simulink model "GradientAscent"  (R2020b)
settings: Solver=FixedStepDiscrete  StartTime=0.0  StopTime=150  FixedStep=Ts  RelTol=1e-3
PreLoadFcn:
  | ROSconfig
  | wptsSignalSetup
InitFcn:
  | configParameters
StartFcn:
  | gazeboSetup
StopFcn:
  | gazeboReset
  | goalreset
  | loadResults
model workspace (MAT data in the model file):
  goalpoints = Simulink.Signal
  goalpoints.DataType = 'auto'
  goalpoints.Dimensions = -1
  goalpoints.DimensionsMode = 'auto'
  goalpoints.Complexity = 'auto'
  goalpoints.SampleTime = -1
  goalpoints.SamplingMode = 'auto'
  goals = Simulink.Signal
  goals.DataType = 'auto'
  goals.Dimensions = -1
  goals.DimensionsMode = 'auto'
  goals.Complexity = 'auto'
  goals.SampleTime = -1
  goals.SamplingMode = 'auto'
  idx = 1
  y = Simulink.Parameter
  y.DataType = 'auto'
  y.Dimensions = [0 0]
values from neighbouring files (symbols this model uses):
  distThresh = .875    (= 0.875)    [GradientAscentMetrics.m]
  m = [m; i*(2*pi/M)]    [SensorArrangementPlots.m]    (also in sensorArrayTesting.m = [0;0;1.2566;2.5133;3.7699;5.0265])
  mag = 2    [GradientAscentMetrics.m]
  sensorDist = 1    [GradientAscentMetrics.m]
undefined symbols (not defined in the file or in its folder): angmax, Angular, concDetectionAccuracy, DiscIntNeverNeededParam, distError, get, init, initX, initY, Kd, Ki, Kp, Linear, MaxC, N, n, OffsetY, PlumeD, Res, ResX, ResY, sourceAccuracy, Tmax, vmax, wgain
libraries: simulink x14, dspswit3 x4, robotlib x3, sm_lib x2, dspsnks4 x2, nesl_utility x1, dspindex x1, mobileRoboticsLib x1
PauseFcn:
  | gazeboPause
settings Model: OrderedModelArguments=off  Creator=ty  LastModifiedBy=Tyreeses'
settings SolverCC: AlgebraicLoopSolver=LineSearch
settings DataIOCC: ExternalInput=[r, b]  SaveFormat=Array  SaveState=on  InspectSignalLogs=on  ReturnWorkspaceOutputs=off  StateSaveName=wpts
settings DebuggingCC: ArithmeticOperatorsInVariantConditions=warning
settings SFSimCC: SimUseLocalCustomCode=off  CustomCodeUndefinedFunction=UseInterfaceOnly
settings RTWCC: RTWUseLocalCustomCode=off
settings SimMechanicsCC: VisOnUpdateDiagram=on  VisDuringSimulation=on  DefaultBodyColor=[.877 0 0]
settings ExplorerConfigSet: SimMechanicsOpenEditorOnUpdate=off  InternalSimMechanicsExplorerSettings="<ExplorerConfiguration><canonicalview>default</canonicalview><AnimationSetting><BasePlaybackSpeed>1.0</BasePlaybackSpeed><PlaybackSpeedFactor>4.0</PlaybackSpeedFactor></AnimationSetting><TilePanel><TileInfo><Tiles Columns=\"2\" Count=\"4\" Rows=\"2\"><Column Weight=\"0.5\"/><Column Weight=\"0.5\"/><Row Weight=\"0.5\"/><Row Weight=\"0.5\"/><Tile Height=\"1\" Width=\"1\" X=\"0\" Y=\"0\"/><Tile Height=\"1\" Width=\"1\" X=\"0\" Y=\"1\"/><Tile Height=\"1\" Width=\"1\" X=\"1\" Y=\"0\"/><Tile Height=\"1\" Width=\"1\" X=\"1\" Y=\"1\"/></Tiles></TileInfo><SceneInfo><SceneViewer><BGColor><R>0.60000002384185791</R><G>0.60000002384185791</G><B>0.60000002384185791</B></BGColor><Camera><DoPerspective>off</DoPerspective><Position><X>0.523539858098702515</X><Y>-0.526832295844210763</Y><Z>1.31558763938248235</Z></Position><Center><X>0.523539858098702515</X><Y>-0.526832295844210763</Y><Z>0.315587639382482354</Z></Center><Up><X>0</X><Y>1</Y><Z>-0</Z></Up><ViewLimDist>1</ViewLimDist><YLim>8.09056691591361421</YLim><XLim>11.4549610789668002</XLim></Camera></SceneViewer><SceneViewer><BGColor><R>0.60000002384185791</R><G>0.60000002384185791</G><B>0.60000002384185791</B></BGColor><Camera><DoPerspective>off</DoPerspective><Position><X>-1.00000000034924597</X><Y>-0.123102183445061519</Y><Z>0.275798201199813964</Z></Position><Center><X>-3.49245965480804443e-10</X><Y>-0.123102183445061519</Y><Z>0.275798201199813964</Z></Center><Up><X>0</X><Y>0</Y><Z>1</Z></Up><ViewLimDist>1</ViewLimDist><YLim>3.47753295219900371</YLim><XLim>4.92363576400452985</XLim></Camera></SceneViewer><SceneViewer><BGColor><R>0.60000002384185791</R><G>0.60000002384185791</G><B>0.60000002384185791</B></BGColor><Camera><DoPerspective>off</DoPerspective><Position><X>0.692144908773628886</X><Y>-0.692774488443842151</Y><Z>0.641997243049143074</Z></Position><Center><X>0.114794639584003433</X><Y>-0.115424219254216046</Y><Z>0.0646469738595174259</Z></Center><Up><X>-0.408248290463863073</X><Y>0.408248290463863073</Y><Z>0.816496580927726145</Z></Up><ViewLimDist>1</ViewLimDist><YLim>6.0070720394774666</YLim><XLim>8.50506239252750262</XLim></Camera></SceneViewer><SceneViewer><BGColor><R>0.60000002384185791</R><G>0.60000002384185791</G><B>0.60000002384185791</B></BGColor><Camera><DoPerspective>off</DoPerspective><Position><X>0.0489598554332313918</X><Y>-0.287272213681231237</Y><Z>1.31558770067272501</Z></Position><Center><X>0.0489598554332313918</X><Y>-0.287272213681231237</Y><Z>0.315587700672725013</Z></Center><Up><X>0</X><Y>1</Y><Z>-0</Z></Up><ViewLimDist>1</ViewLimDist><YLim>2.42704539801906094</YLim><XLim>3.4363118011556999</XLim></Camera></SceneViewer></SceneInfo></TilePanel><MechEditorPanel><Cameras><Camera><Id>Camera1</Id><Value><Name>TopCamera1</Name><NativeCamera><PositionKeyframeSet><Keyframe><Time>+0.0000000000000000e+00</Time><Value><X>+2.1442706964244174e-01</X><Y>+2.3082412087368320e-01</Y><Z>+8.5801428178680403e+00</Z></Value></Keyframe></PositionKeyframeSet><CenterKeyframeSet><Keyframe><Time>+0.0000000000000000e+00</Time><Value><X>+1.7666087274208450e-01</X><Y>+1.6219238056249624e-01</Y><Z>+3.9566976367888529e-01</Z></Value></Keyframe></CenterKeyframeSet><UpVectorKeyframeSet><Keyframe><Time>+0.0000000000000000e+00</Time><Value><X>-1.4536948631457236e-02</X><Y>+9.9985973958876295e-01</Y><Z>-8.3173477730344968e-03</Z></Value></Keyframe></UpVectorKeyframeSet></NativeCamera></Value></Camera></Cameras><GfxPanelCameraMap/><VideoCreator><PlaybackSpeedRatio>1.0</PlaybackSpeedRatio><FrameRate>30</FrameRate><VideoFormat>Motion JPEG AVI</VideoFormat><FrameSize>auto</FrameSize></VideoCreator></MechEditorPanel></ExplorerConfiguration>"

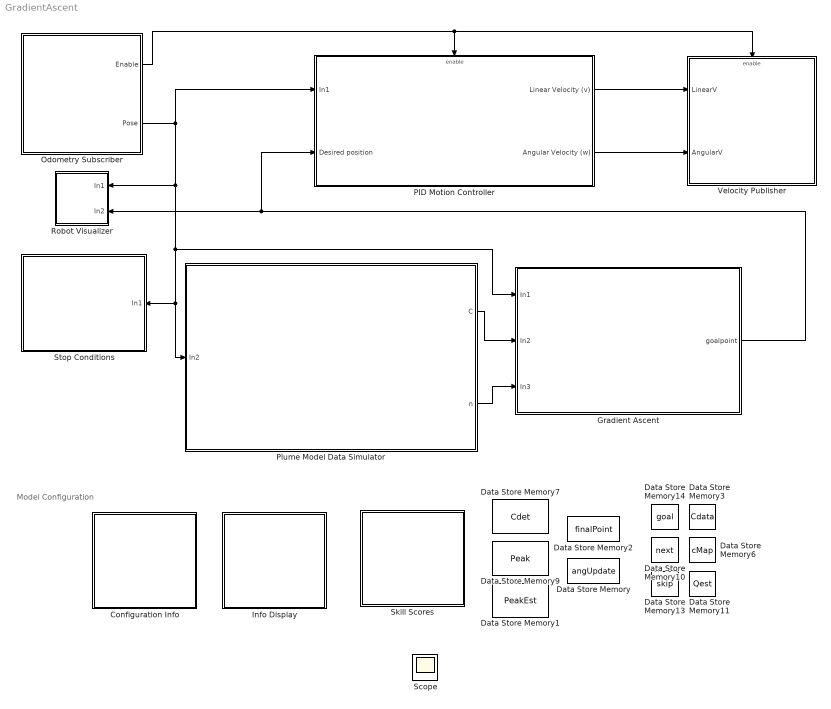
== system GradientAscent ==
  note: Model Configuration
  Configuration Info : Subsystem
  Data Store Memory : DataStoreMemory  DataStoreName=angUpdate  ReadBeforeWriteMsg=warning  WriteAfterWriteMsg=warning  WriteAfterReadMsg=warning  ShowAdditionalParam=off
  Data Store Memory1 : DataStoreMemory  DataStoreName=PeakEst  ReadBeforeWriteMsg=warning  WriteAfterWriteMsg=warning  WriteAfterReadMsg=warning  InitialValue=[(initX) (initY)]  VectorParams1D=off  ShowAdditionalParam=off
  Data Store Memory10 : DataStoreMemory  DataStoreName=next  ReadBeforeWriteMsg=warning  WriteAfterWriteMsg=warning  WriteAfterReadMsg=warning  ShowAdditionalParam=off
  Data Store Memory11 : DataStoreMemory  DataStoreName=Qest  ReadBeforeWriteMsg=warning  WriteAfterWriteMsg=warning  WriteAfterReadMsg=warning  ShowAdditionalParam=off
  Data Store Memory13 : DataStoreMemory  DataStoreName=skip  ReadBeforeWriteMsg=warning  WriteAfterWriteMsg=warning  WriteAfterReadMsg=warning  ShowAdditionalParam=off
  Data Store Memory14 : DataStoreMemory  DataStoreName=goal  ReadBeforeWriteMsg=warning  WriteAfterWriteMsg=warning  WriteAfterReadMsg=warning  VectorParams1D=off  ShowAdditionalParam=off
  Data Store Memory2 : DataStoreMemory  DataStoreName=finalPoint  ReadBeforeWriteMsg=warning  WriteAfterWriteMsg=warning  WriteAfterReadMsg=warning  ShowAdditionalParam=off
  Data Store Memory3 : DataStoreMemory  DataStoreName=Cdata  ReadBeforeWriteMsg=warning  WriteAfterWriteMsg=warning  WriteAfterReadMsg=warning  InitialValue=ones(N+1,1)  ShowAdditionalParam=off  OutDataTypeStr=double
  Data Store Memory6 : DataStoreMemory  DataStoreName=cMap  ReadBeforeWriteMsg=warning  WriteAfterWriteMsg=warning  WriteAfterReadMsg=warning  InitialValue=zeros(50,500)  VectorParams1D=off  ShowAdditionalParam=off
  Data Store Memory7 : DataStoreMemory  DataStoreName=Cdet  ReadBeforeWriteMsg=warning  WriteAfterWriteMsg=warning  WriteAfterReadMsg=warning  ShowAdditionalParam=off
  Data Store Memory9 : DataStoreMemory  DataStoreName=Peak  ReadBeforeWriteMsg=warning  WriteAfterWriteMsg=warning  WriteAfterReadMsg=warning  InitialValue=[0 0]  ShowAdditionalParam=off
  Gradient Ascent : Subsystem
  Info Display : Subsystem
  Odometry Subscriber : Subsystem
  PID Motion Controller : Subsystem
  Plume Model Data Simulator : Subsystem
  Robot Visualizer : Subsystem
  Skill Scores : Subsystem
  Stop Conditions : Subsystem
  Velocity Publisher : Subsystem
  Scope : Scope
  wires:
  Odometry Subscriber/1(Enable) -> Velocity Publisher/Enable, PID Motion Controller/Enable
  PID Motion Controller/1(Linear Velocity (v)) -> Velocity Publisher/1(LinearV)
  PID Motion Controller/2(Angular Velocity (w)) -> Velocity Publisher/2(AngularV)
  Gradient Ascent/1(goalpoint) -> PID Motion Controller/2(Desired position), Robot Visualizer/2(In2)
  Plume Model Data Simulator/1(C) -> Gradient Ascent/2(In2)
  Plume Model Data Simulator/2(n) -> Gradient Ascent/3(In3)
  Odometry Subscriber/2(Pose) -> Plume Model Data Simulator/1(In2), Stop Conditions/1(In1), Gradient Ascent/1(In1), Robot Visualizer/1(In1), PID Motion Controller/1(In1)

== system GradientAscent/Configuration Info ==
  note: Nodes :
      | Publishers:
      | /sim_p3at/cmd_vel
      | /toggle_led
      | Subscribers:
      | /sim_p3at/odom
      | Messages:
      | geometry_msgs/Twist
      | std_msgs/Empty
  note: Startup Programs :
      | roscore
      | roslaunch nre_p3at p3at.gazebo.launch (starts Gazebo and /sim_p3at Nodes)
      | Arduino: ledtest3.ino
      | rosrun rosserial_python serial_node.py /dev/ttyACM0
      | MATLAB: (Simulink project)
  note: SS Parameters :
      | Expansion Constant: 2
  note: Plume Parameters :
      |
      | Diffusion constant (m2/s): c_diff = .8
      |
      | Advection velocity values (m/s): ux = 0 uy = 0 uz = 0.2
      |
      | Simulation Time (seconds): T = 10
      |
      | Domain dimensions (meters): L = 50 B = 50 H = 5
  "Counter " : Subsystem  Commented=on
  Floating Scope : Scope  Commented=on
      settings: Floating=on
  MechanismConfiguration : sm_lib/Utilities/Mechanism Configuration  UniformGravity=Constant  GravityVector=[0 0 -9.80665]  GravityUnits=m/s^2  LinearizationDelta=0.01
  Solver Configuration : nesl_utility/Solver Configuration  PhysicalDomain=network_engine_domain  SubClassName=solver  LeftPortType=input  RightPortType=generic  Accelerate=off  Tones=[]  Harmonics=[]  SimulateNoise=off  Profile=off  UseLocalSampling=off  EnableSwitchedLinearOptims=on  FrequencyDomain=off  UseCCode=off  RelTol=0.001  AbsTol=1e-06  MinStep=1e-09  ToWorkspace=off  RevertToSquareIcSolve=off  NumHomotopyIterations=100  PhasorMode=off  PhasorModeNumHarmonics=1  DoDC=on  ResidualTolerance=1e-09  UseLocalSolver=on  LocalSolverChoice=NE_BACKWARD_EULER_ADVANCER  LocalSolverSampleTime=Ts  DoFixedCost=on  MaxNonlinIter=3  MaxModeIter=2  LinearAlgebra=Sparse  DelaysMemoryBudget=1024  AutomaticFiltering=on  FilteringTimeConstant=0.01
  World : sm_lib/Frames and Transforms/World Frame
  connections:
  MechanismConfiguration/RConn1 -- World/RConn1 -- Solver Configuration/RConn1

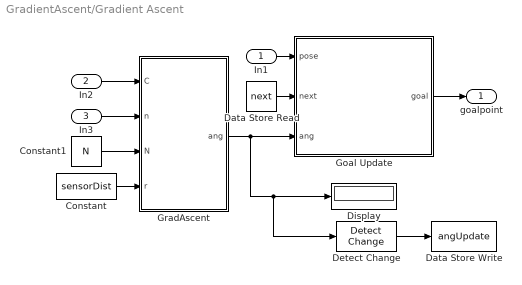
== system GradientAscent/Gradient Ascent ==
  In1 : Inport
  In2 : Inport  Port=2
  In3 : Inport  Port=3
  Constant : Constant  Value=sensorDist
  Constant1 : Constant  Value=N
  Data Store Read : DataStoreRead  DataStoreName=next
  Data Store Write : DataStoreWrite  DataStoreName=angUpdate
  Detect Change : simulink/Logic and Bit Operations/Detect Change  vinit=1.514  OutDataTypeStr=boolean
  Display : Display
  Goal Update : Subsystem
  GradAscent : MATLAB Function  TreatAsAtomicUnit=on
  goalpoint : Outport  VectorParamsAs1DForOutWhenUnconnected=off
  wires:
  In1/1 -> Goal Update/1(pose)
  In3/1 -> GradAscent/2(n)
  GradAscent/1(ang) -> Detect Change/1, Display/1, Goal Update/3(ang)
  Goal Update/1(goal) -> goalpoint/1
  Data Store Read/1 -> Goal Update/2(next)
  Constant/1 -> GradAscent/4(r)
  Constant1/1 -> GradAscent/3(N)
  Detect Change/1 -> Data Store Write/1
  In2/1 -> GradAscent/1(C)

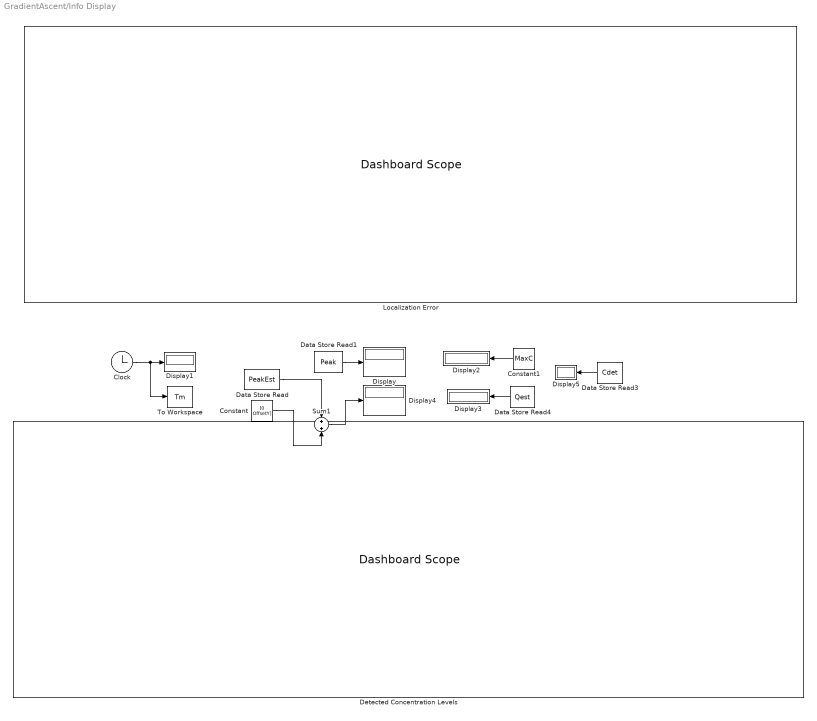
== system GradientAscent/Info Display ==
  Clock : Clock
      settings: Decimation=2
  Constant : Constant  Value=[0 OffsetY]
  Constant1 : Constant  Value=MaxC
  Data Store Read : DataStoreRead  DataStoreName=PeakEst
  Data Store Read1 : DataStoreRead  DataStoreName=Peak
  Data Store Read3 : DataStoreRead  DataStoreName=Cdet
  Data Store Read4 : DataStoreRead  DataStoreName=Qest
  Detected Concentration Levels : DashboardScope  ShowInitialText=off  Ymin=0  Ymax=1000
  Display{,1..5} (6 alike) : Display
  Localization Error : DashboardScope  Ymin=0  Ymax=1.25  LegendPosition=Hide
  Sum1 : Sum
  To Workspace : ToWorkspace  VariableName=Tm  SampleTime=-1
  wires:
  Data Store Read1/1 -> Display/1
  Data Store Read/1 -> Sum1/1
  Data Store Read4/1 -> Display3/1
  Constant1/1 -> Display2/1
  Clock/1 -> To Workspace/1, Display1/1
  Data Store Read3/1 -> Display5/1
  Constant/1 -> Sum1/2
  Sum1/1 -> Display4/1

== system GradientAscent/Odometry Subscriber ==
  Odom Conversion : Subsystem
  Subscribe1 : robotlib/Subscribe  topicSource=Select from ROS network  topic=/sim_p3at/odom  messageType=nav_msgs/Odometry  SampleTime=-1  legacyBusStruct=off  messageQueueLength=51
  Enable : Outport  VectorParamsAs1DForOutWhenUnconnected=off
  Pose : Outport  Port=2  VectorParamsAs1DForOutWhenUnconnected=off
  wires:
  Subscribe1/1 -> Enable/1
  Subscribe1/2 -> Odom Conversion/1(In1)
  Odom Conversion/1(pose) -> Pose/1

== system GradientAscent/PID Motion Controller ==
  In1 : Inport
  Desired position : Inport  Port=2
  Enable : EnablePort
  Constant3 : Constant  Value=0
  Demux : Demux  Outputs=3
  PID Calculations : Subsystem
  Switch1 : Switch  Criteria=u2 ~= 0
  Linear Velocity (v) : Outport  VectorParamsAs1DForOutWhenUnconnected=off
  Angular Velocity (w) : Outport  Port=2  VectorParamsAs1DForOutWhenUnconnected=off
  wires:
  Switch1/1 -> Angular Velocity (w)/1
  Constant3/1 -> Switch1/1
  Demux/1 -> PID Calculations/3(x)
  Demux/2 -> PID Calculations/2(y)
  Demux/3 -> PID Calculations/4(theta)
  PID Calculations/3(w) -> Switch1/3
  In1/1 -> Demux/1
  PID Calculations/2(next) -> Switch1/2
  Desired position/1 -> PID Calculations/1(SP)  "SP"
  PID Calculations/1(v) -> Linear Velocity (v)/1

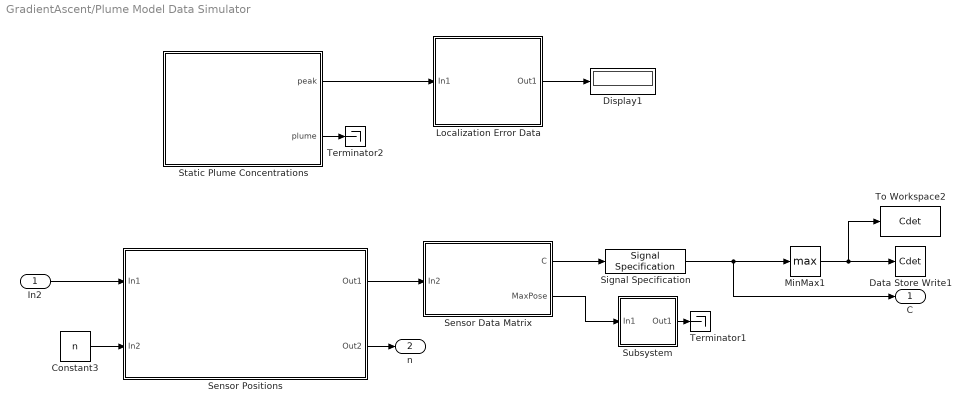
== system GradientAscent/Plume Model Data Simulator ==
  In2 : Inport
  Constant3 : Constant  Value=n
  Data Store Write1 : DataStoreWrite  DataStoreName=Cdet
  Display1 : Display
  Localization Error Data : Subsystem
  MinMax1 : MinMax  Function=max
  Sensor Data Matrix : Subsystem
  Sensor Positions : Subsystem
  Signal Specification : SignalSpecification  OutDataTypeStr=double  SampleTime=.01
  Static Plume Concentrations : Subsystem
  Subsystem : Subsystem
  Terminator1 : Terminator
  Terminator2 : Terminator
  To Workspace2 : ToWorkspace  VariableName=Cdet  SaveFormat=Timeseries  SampleTime=-1
  C : Outport  VectorParamsAs1DForOutWhenUnconnected=off
  n : Outport  Port=2  VectorParamsAs1DForOutWhenUnconnected=off
  wires:
  Sensor Positions/1(Out1) -> Sensor Data Matrix/1(In2)
  MinMax1/1 -> To Workspace2/1, Data Store Write1/1
  Sensor Data Matrix/1(C) -> Signal Specification/1
  Signal Specification/1 -> C/1, MinMax1/1
  In2/1 -> Sensor Positions/1(In1)
  Constant3/1 -> Sensor Positions/2(In2)
  Static Plume Concentrations/1(peak) -> Localization Error Data/1(In1)
  Static Plume Concentrations/2(plume) -> Terminator2/1
  Localization Error Data/1(Out1) -> Display1/1
  Sensor Data Matrix/2(MaxPose) -> Subsystem/1(In1)
  Subsystem/1(Out1) -> Terminator1/1
  Sensor Positions/2(Out2) -> n/1

== system GradientAscent/Robot Visualizer ==
  In1 : Inport
  In2 : Inport  Port=2
  Constant1 : Constant
  Current Origin : dspindex/Variable Selector  NumInputs=1  rowsOrCols=Rows  IdxMode=Variable  Elements=[1 3]  ZerOneIdxMode=One-based  errmode=Clip Index  FillMode=off  FillValues=0
  Data Store Read : DataStoreRead  DataStoreName=next
  Data Store Write : DataStoreWrite  DataStoreName=PeakEst
  Robot Visualizer : mobileRoboticsLib/Environments/Robot Visualizer  Priority=99  robotRadius=.34  mapName=gasMap  showTrajectory=on  hasWaypoints=on  hasLidar=off  sensorOffset=[ 0 0 ]  scanAngles=0  hasObjDetector=off  objDetectorOffset=[ 0,0 ]  objDetectorAngle=0  objDetectorFOV=0  objDetectorMaxRange=0  objectColors=[1,0,0;0,1,0;0,0,1]  objectMarkers='s'
  To Workspace : ToWorkspace  VariableName=goalpoints  SampleTime=-1
      settings: Save2DSignal=2-D array (concatenate along first dimension)
  Triggered To Workspace : dspsnks4/Triggered To Workspace  TriggerType=Rising edge  VariableName=pathUpdates  Buffer=1000  Save2DMode=3-D array (concatenate along third dimension)
      settings: SourceProductBaseCode=DS  FixptAsFi=off
  wires:
  In1/1 -> Robot Visualizer/1
  In2/1 -> To Workspace/1, Current Origin/1, Data Store Write/1, Robot Visualizer/2
  Data Store Read/1 -> Triggered To Workspace/Trigger
  Constant1/1 -> Current Origin/2
  Current Origin/1 -> Triggered To Workspace/1

== system GradientAscent/Skill Scores ==
  Location Estimate (SL) : Subsystem
  Source Estimate (SQ) : Subsystem

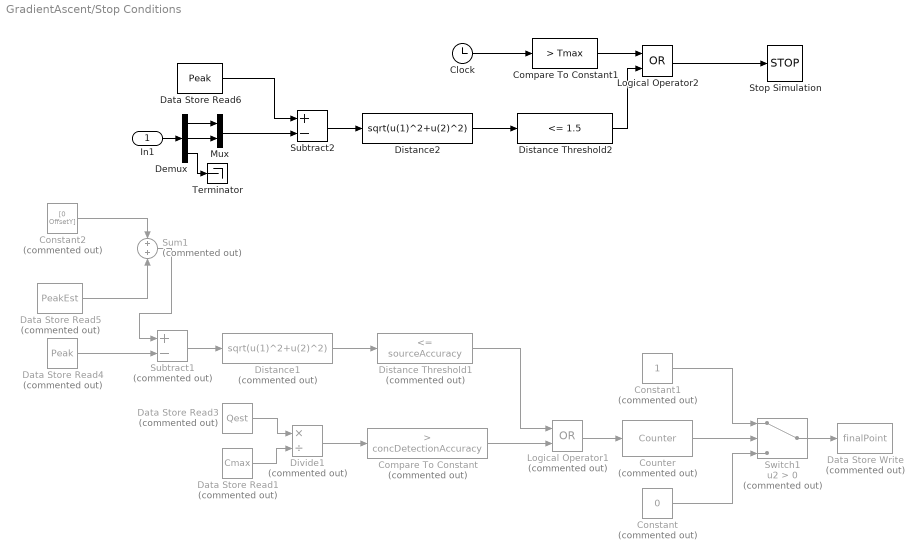
== system GradientAscent/Stop Conditions ==
  In1 : Inport
  Clock : Clock
  Compare To Constant : simulink/Logic and Bit Operations/Compare To Constant  Commented=on  relop=>  const=concDetectionAccuracy  OutDataTypeStr=boolean
  Compare To Constant1 : simulink/Logic and Bit Operations/Compare To Constant  relop=>  const=Tmax  OutDataTypeStr=boolean
  Constant : Constant  Commented=on  Value=0
  Constant1 : Constant  Commented=on
  Constant2 : Constant  Commented=on  Value=[0 OffsetY]
  Counter : dspswit3/Counter  Commented=on  Direction=Up  CountEvent=Rising edge  CounterSize=User defined  MaxCount=255  InitialCount=0  Output=Count  HitValue=32  ResetInput=off  SamplesPerFrame=1  Ts=1  CntDtype=double  HitDtype=Logical
  Data Store Read1 : DataStoreRead  Commented=on  DataStoreName=Cmax
  Data Store Read3 : DataStoreRead  Commented=on  DataStoreName=Qest
  Data Store Read4 : DataStoreRead  Commented=on  DataStoreName=Peak
  Data Store Read5 : DataStoreRead  Commented=on  DataStoreName=PeakEst
  Data Store Read6 : DataStoreRead  DataStoreName=Peak
  Data Store Write : DataStoreWrite  Commented=on  DataStoreName=finalPoint
  Demux : Demux  Outputs=3
  Distance Threshold1 : simulink/Logic and Bit Operations/Compare To Constant  Commented=on  relop=<=  const=sourceAccuracy  OutDataTypeStr=boolean
  Distance Threshold2 : simulink/Logic and Bit Operations/Compare To Constant  relop=<=  const=1.5  OutDataTypeStr=boolean
  Distance1 : Fcn  Commented=on  Expr=sqrt(u(1)^2+u(2)^2)
  Distance2 : Fcn  Expr=sqrt(u(1)^2+u(2)^2)
  Divide1 : Product  Commented=on  Inputs=*/
  Logical Operator1 : Logic  Commented=on  Operator=OR  AllPortsSameDT=off  OutDataTypeStr=boolean
  Logical Operator2 : Logic  Operator=OR  AllPortsSameDT=off  OutDataTypeStr=boolean
  Mux : Mux  Inputs=2
  Stop Simulation : Stop
  Subtract1 : Sum  Commented=on  Inputs=+-
  Subtract2 : Sum  Inputs=+-
  Sum1 : Sum  Commented=on
  Switch1 : Switch  Commented=on  Criteria=u2 > Threshold
  Terminator : Terminator
  wires:
  Logical Operator1/1 -> Counter/1
  Compare To Constant/1 -> Logical Operator1/2
  Data Store Read3/1 -> Divide1/1
  Data Store Read5/1 -> Sum1/2
  Subtract1/1 -> Distance1/1
  Distance Threshold1/1 -> Logical Operator1/1
  Data Store Read4/1 -> Subtract1/2
  Data Store Read1/1 -> Divide1/2
  Distance1/1 -> Distance Threshold1/1
  Divide1/1 -> Compare To Constant/1
  Data Store Read6/1 -> Subtract2/1
  Subtract2/1 -> Distance2/1
  Distance2/1 -> Distance Threshold2/1
  Distance Threshold2/1 -> Logical Operator2/2
  Constant1/1 -> Switch1/1
  Constant/1 -> Switch1/3
  Counter/1 -> Switch1/2
  Switch1/1 -> Data Store Write/1
  In1/1 -> Demux/1
  Demux/1 -> Mux/1
  Demux/2 -> Mux/2
  Mux/1 -> Subtract2/2
  Demux/3 -> Terminator/1
  Constant2/1 -> Sum1/1
  Sum1/1 -> Subtract1/1
  Compare To Constant1/1 -> Logical Operator2/1
  Clock/1 -> Compare To Constant1/1
  Logical Operator2/1 -> Stop Simulation/1

== system GradientAscent/Velocity Publisher ==
  LinearV : Inport
  AngularV : Inport  Port=2
  Enable : EnablePort
  Blank Message : robotlib/Blank Message  SourceLibraryInfo=This block requires Robotics System Toolbox  messageType=geometry_msgs/Twist  SampleTime=-1
  Bus Assignment : BusAssignment  DialogController=Simulink.DDGSource_BusAssignment  AssignedSignals=Linear.X,Angular.Z
  Publish1 : robotlib/Publish  SourceLibraryInfo=This block requires Robotics System Toolbox  topicSource=Select from ROS network  topic=/sim_p3at/cmd_vel  messageType=geometry_msgs/Twist  messageQueueLength=105
  wires:
  AngularV/1 -> Bus Assignment/3
  Bus Assignment/1 -> Publish1/1
  LinearV/1 -> Bus Assignment/2
  Blank Message/1 -> Bus Assignment/1

== system GradientAscent/Configuration Info/Counter  ==
  In1 : Inport
  Counter : dspswit3/Counter  Direction=Up  CountEvent=Non-zero sample  CounterSize=User defined  MaxCount=255  InitialCount=0  Output=Count  HitValue=32  ResetInput=off  SamplesPerFrame=1  Ts=1  CntDtype=single  HitDtype=Logical
  Counter1 : dspswit3/Counter  Direction=Up  CountEvent=Rising edge  CounterSize=User defined  MaxCount=255  InitialCount=0  Output=Count  HitValue=32  ResetInput=off  SamplesPerFrame=1  Ts=1  CntDtype=double  HitDtype=Logical
  Detect Increase : simulink/Logic and Bit Operations/Detect Increase  vinit=0.0  OutDataTypeStr=boolean
  Out1 : Outport  VectorParamsAs1DForOutWhenUnconnected=off
  wires:
  In1/1 -> Counter/1
  Counter/1 -> Detect Increase/1
  Detect Increase/1 -> Counter1/1
  Counter1/1 -> Out1/1

== system GradientAscent/Gradient Ascent/Goal Update ==
  pose : Inport
  next : Inport  Port=2
  ang : Inport  Port=3
  Goal Update : Subsystem
  Goal Update Conditions : Subsystem
  Initialize Goal : Subsystem
  Skip Conditions : Subsystem
  goal : Outport  VectorParamsAs1DForOutWhenUnconnected=off
  wires:
  pose/1 -> Goal Update/1(In2)
  ang/1 -> Goal Update/2(In3)
  Goal Update Conditions/1(Out1) -> Goal Update/Enable
  next/1 -> Skip Conditions/1(In1)
  Initialize Goal/1(goal) -> Goal Update Conditions/1(In1), goal/1
  Goal Update/1(Out2) -> Initialize Goal/1(In1)

== system GradientAscent/Odometry Subscriber/Odom Conversion ==
  In1 : Inport
  Bus Selector3 : BusSelector  OutputSignals=Pose.Pose.Position.X,Pose.Pose.Position.Y,Pose.Pose.Orientation.X,Pose.Pose.Orientation.Y,Pose.Pose.Orientation.Z,Pose.Pose.Orientation.W
  Conversion : MATLAB Function  TreatAsAtomicUnit=on
  Mux : Mux  Inputs=3
  pose : Outport  VectorParamsAs1DForOutWhenUnconnected=off
  wires:
  In1/1 -> Bus Selector3/1
  Bus Selector3/3 -> Conversion/1(x)  "<X>"
  Bus Selector3/4 -> Conversion/2(y)  "<Y>"
  Bus Selector3/5 -> Conversion/3(z)  "<Z>"
  Bus Selector3/6 -> Conversion/4(w)  "<W>"
  Bus Selector3/2 -> Mux/2  "<Y>"
  Bus Selector3/1 -> Mux/1  "<X>"
  Mux/1 -> pose/1  "pose"
  Conversion/1(yaw) -> Mux/3

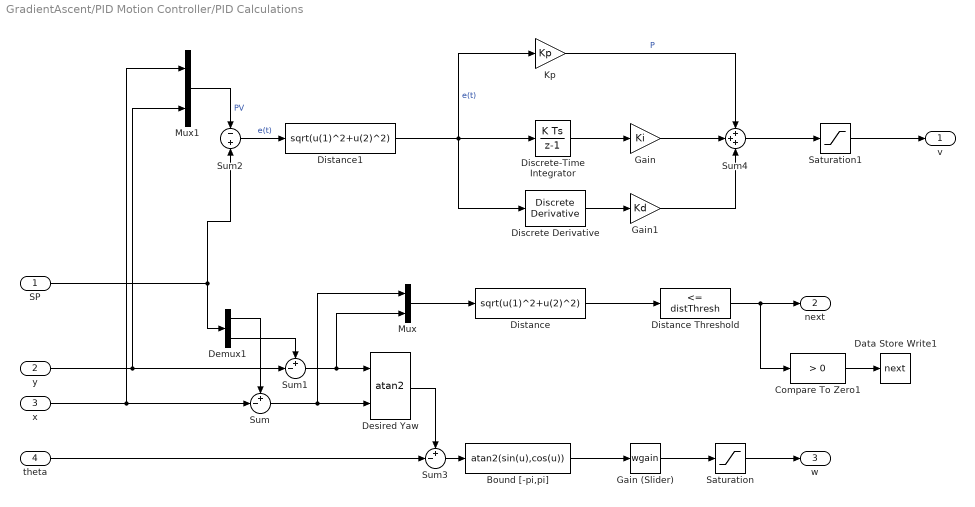
== system GradientAscent/PID Motion Controller/PID Calculations ==
  SP : Inport
  y : Inport  Port=2
  x : Inport  Port=3
  theta : Inport  Port=4
  Bound [-pi,pi] : Fcn  Expr=atan2(sin(u),cos(u))
  Compare To Zero1 : simulink/Logic and Bit Operations/Compare To Zero  relop=>  OutDataTypeStr=boolean
  Data Store Write1 : DataStoreWrite  DataStoreName=next
  Demux1 : Demux  Outputs=2
  Desired Yaw : Trigonometry  Operator=atan2
  Discrete Derivative : simulink/Discrete/Discrete Derivative  gainval=1  ICPrevScaledInput=0.0  OutMin=[]  OutMax=[]  OutDataType=fixdt(1, 16)  OutScaling=2^-10  DoSatur=off
  Discrete-Time Integrator : DiscreteIntegrator  gainval=1  SampleTime=-1  ICPrevOutput=DiscIntNeverNeededParam  ICPrevScaledInput=DiscIntNeverNeededParam
  Distance : Fcn  Expr=sqrt(u(1)^2+u(2)^2)
  Distance Threshold : simulink/Logic and Bit Operations/Compare To Constant  relop=<=  const=distThresh  OutDataTypeStr=boolean
  Distance1 : Fcn  Expr=sqrt(u(1)^2+u(2)^2)
  Gain : Gain  Gain=Ki
  Gain (Slider) : simulink/Math Operations/Slider Gain  gain=wgain  low=1  high=10
  Gain1 : Gain  Gain=Kd
  Kp : Gain  Gain=Kp
  Mux : Mux  Inputs=2
  Mux1 : Mux  Inputs=2
  Saturation : Saturate  UpperLimit=angmax  LowerLimit=-angmax
  Saturation1 : Saturate  UpperLimit=vmax  LowerLimit=-.5
  Sum : Sum  Inputs=+-|
  Sum1 : Sum  Inputs=+-|
  Sum2 : Sum  Inputs=-+
  Sum3 : Sum  Inputs=+-|
  Sum4 : Sum  Inputs=+++
  v : Outport  VectorParamsAs1DForOutWhenUnconnected=off
  next : Outport  Port=2  VectorParamsAs1DForOutWhenUnconnected=off
  w : Outport  Port=3  VectorParamsAs1DForOutWhenUnconnected=off
  wires:
  theta/1 -> Sum3/2
  Desired Yaw/1 -> Sum3/1
  Sum/1 -> Desired Yaw/2, Mux/1
  Gain (Slider)/1 -> Saturation/1
  Saturation/1 -> w/1
  Sum3/1 -> Bound [-pi,pi]/1
  Mux1/1 -> Sum2/1  "PV"
  Kp/1 -> Sum4/1  "P"
  Distance1/1 -> Kp/1, Discrete-Time Integrator/1, Discrete Derivative/1  "e(t)"
  Discrete-Time Integrator/1 -> Gain/1
  Demux1/1 -> Sum/1
  Demux1/2 -> Sum1/1
  Sum1/1 -> Desired Yaw/1, Mux/2
  SP/1 -> Demux1/1, Sum2/2
  y/1 -> Mux1/2, Sum1/2
  x/1 -> Mux1/1, Sum/2
  Distance/1 -> Distance Threshold/1
  Mux/1 -> Distance/1
  Bound [-pi,pi]/1 -> Gain (Slider)/1
  Sum2/1 -> Distance1/1  "e(t)"
  Gain/1 -> Sum4/2
  Sum4/1 -> Saturation1/1
  Discrete Derivative/1 -> Gain1/1
  Gain1/1 -> Sum4/3
  Saturation1/1 -> v/1
  Distance Threshold/1 -> Compare To Zero1/1, next/1
  Compare To Zero1/1 -> Data Store Write1/1

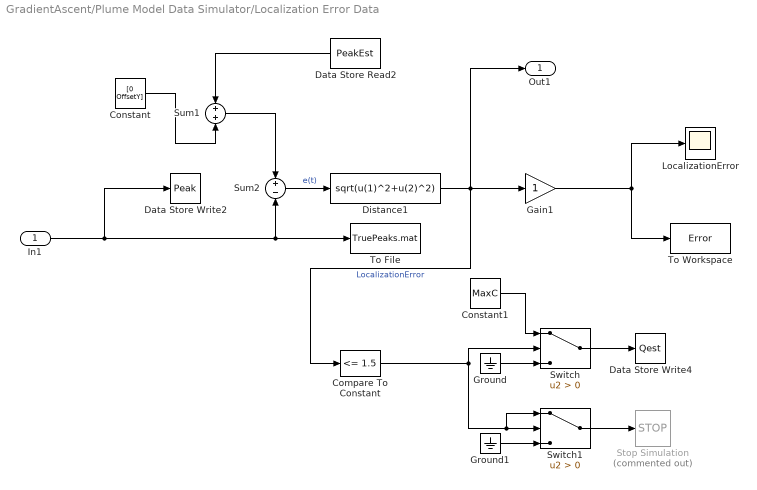
== system GradientAscent/Plume Model Data Simulator/Localization Error Data ==
  In1 : Inport
  Compare To Constant : simulink/Logic and Bit Operations/Compare To Constant  relop=<=  const=1.5  OutDataTypeStr=boolean
  Constant : Constant  Value=[0 OffsetY]
  Constant1 : Constant  Value=MaxC
  Data Store Read2 : DataStoreRead  DataStoreName=PeakEst
  Data Store Write2 : DataStoreWrite  DataStoreName=Peak
  Data Store Write4 : DataStoreWrite  DataStoreName=Qest
  Distance1 : Fcn  Expr=sqrt(u(1)^2+u(2)^2)
  Gain1 : Gain
  Ground : Ground
  Ground1 : Ground
  LocalizationError : Scope
  Stop Simulation : Stop  Commented=on
  Sum1 : Sum
  Sum2 : Sum  Inputs=+-
  Switch : Switch  Criteria=u2 > Threshold
  Switch1 : Switch  Criteria=u2 > Threshold
  To File : ToFile  Filename=TruePeaks.mat  MatrixName=ActualPeaks
      settings: Decimation=2
  To Workspace : ToWorkspace  VariableName=Error  SaveFormat=Timeseries  SampleTime=-1
  Out1 : Outport  VectorParamsAs1DForOutWhenUnconnected=off
  wires:
  Sum2/1 -> Distance1/1  "e(t)"
  Data Store Read2/1 -> Sum1/1
  Distance1/1 -> Out1/1, Compare To Constant/1, Gain1/1  "LocalizationError"
  In1/1 -> Data Store Write2/1, To File/1, Sum2/2
  Constant/1 -> Sum1/2
  Sum1/1 -> Sum2/1
  Gain1/1 -> To Workspace/1, LocalizationError/1
  Compare To Constant/1 -> Switch1/1, Switch1/2, Switch/2
  Ground/1 -> Switch/3
  Constant1/1 -> Switch/1
  Ground1/1 -> Switch1/3
  Switch1/1 -> Stop Simulation/1
  Switch/1 -> Data Store Write4/1

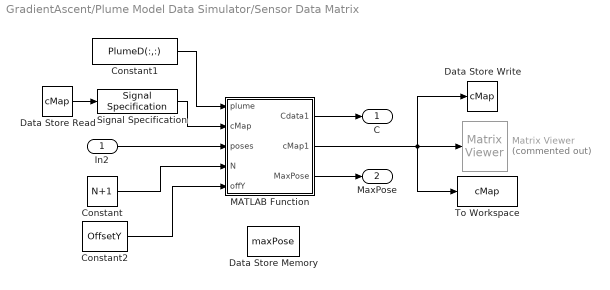
== system GradientAscent/Plume Model Data Simulator/Sensor Data Matrix ==
  In2 : Inport
  Constant : Constant  Value=N+1
  Constant1 : Constant  Value=PlumeD(:,:)
  Constant2 : Constant  Value=OffsetY
  Data Store Memory : DataStoreMemory  DataStoreName=maxPose  ReadBeforeWriteMsg=warning  WriteAfterWriteMsg=warning  WriteAfterReadMsg=warning  InitialValue=init  VectorParams1D=off  ShowAdditionalParam=off  OutDataTypeStr=double
  Data Store Read : DataStoreRead  DataStoreName=cMap
  Data Store Write : DataStoreWrite  DataStoreName=cMap
  MATLAB Function : MATLAB Function  TreatAsAtomicUnit=on
  Matrix Viewer : dspsnks4/Matrix Viewer  Commented=on  ImageParams=off  CMapStr=jet  AxisColorbar=on  AxisParams=off  AxisOrigin=Lower left corner  AxisTickMode=Auto  XTickRange=[0 150]  YTickRange=[0 50]  XLabel=X-axis  YLabel=Y-axis  ZLabel=Concentration  FigPos=get(0,'defaultfigureposition')  AxisZoom=off
      settings: SourceProductBaseCode=DS  YMin=0  YMax=MaxC
  Signal Specification : SignalSpecification  OutDataTypeStr=double  SampleTime=.01
  To Workspace : ToWorkspace  VariableName=cMap  SampleTime=-1
      settings: MaxDataPoints=100
  C : Outport  VectorParamsAs1DForOutWhenUnconnected=off
  MaxPose : Outport  Port=2  VectorParamsAs1DForOutWhenUnconnected=off
  wires:
  Constant/1 -> MATLAB Function/4(N)
  In2/1 -> MATLAB Function/3(poses)
  MATLAB Function/1(Cdata1) -> C/1
  Constant1/1 -> MATLAB Function/1(plume)
  Constant2/1 -> MATLAB Function/5(offY)
  Data Store Read/1 -> Signal Specification/1
  MATLAB Function/2(cMap1) -> To Workspace/1, Data Store Write/1, Matrix Viewer/1
  Signal Specification/1 -> MATLAB Function/2(cMap)
  MATLAB Function/3(MaxPose) -> MaxPose/1

== system GradientAscent/Plume Model Data Simulator/Sensor Positions ==
  In1 : Inport
  In2 : Inport  Port=2
  Radial Sensors : Subsystem
  Sensor Array : Subsystem
  Sensor Center : Subsystem
  Out1 : Outport  VectorParamsAs1DForOutWhenUnconnected=off
  Out2 : Outport  Port=2  VectorParamsAs1DForOutWhenUnconnected=off
  wires:
  In1/1 -> Radial Sensors/1(In1), Sensor Center/1(In2)
  In2/1 -> Radial Sensors/2(In2)
  Sensor Center/1(n) -> Sensor Array/1(In1)
  Sensor Center/2(Out1) -> Sensor Array/2(In2)
  Radial Sensors/1(Out1) -> Sensor Array/3(In3)
  Radial Sensors/2(Out2) -> Sensor Array/4(In4)
  Sensor Array/1(Out2) -> Out1/1
  Sensor Array/2(Out3) -> Out2/1

== system GradientAscent/Plume Model Data Simulator/Static Plume Concentrations ==
  Constant : Constant  Value=OffsetY
  Dynamic Plume Concentration Data : Constant  Value=PlumeD  VectorParams1D=off  OutDataTypeStr=double  LockScale=on
  MATLAB Function : MATLAB Function  TreatAsAtomicUnit=on
  Permute Dimensions1 : PermuteDimensions
  peak : Outport  VectorParamsAs1DForOutWhenUnconnected=off
  plume : Outport  Port=2  VectorParamsAs1DForOutWhenUnconnected=off
  wires:
  Dynamic Plume Concentration Data/1 -> MATLAB Function/1(PlumeD)
  MATLAB Function/1(Plume) -> Permute Dimensions1/1
  Permute Dimensions1/1 -> plume/1
  MATLAB Function/2(Peak) -> peak/1
  Constant/1 -> MATLAB Function/2(OffsetY)

== system GradientAscent/Plume Model Data Simulator/Subsystem ==
  In1 : Inport
  Constant : Constant
  Constant1 : Constant  Value=2
  Selector : Selector  InputPortWidth=2  IndexOptions=Index vector (port)  Indices=1  OutputSizes=1
  Selector2 : Selector  InputPortWidth=2  IndexOptions=Index vector (port)  Indices=1  OutputSizes=1
  Signal Specification1 : SignalSpecification  OutDataTypeStr=double  SampleTime=.01
  Vector Concatenate : Concatenate
  Out1 : Outport  VectorParamsAs1DForOutWhenUnconnected=off
  wires:
  Constant/1 -> Selector/2
  Vector Concatenate/1 -> Out1/1
  Constant1/1 -> Selector2/2
  Selector2/1 -> Vector Concatenate/2
  Signal Specification1/1 -> Selector/1, Selector2/1
  Selector/1 -> Vector Concatenate/1
  In1/1 -> Signal Specification1/1

== system GradientAscent/Skill Scores/Location Estimate (SL) ==
  Data Store Read : DataStoreRead  DataStoreName=Peak
  Data Store Read2 : DataStoreRead  DataStoreName=PeakEst
  Distance : Fcn  Expr=sqrt(u(1)^2+u(2)^2)
  Distance Threshold : simulink/Logic and Bit Operations/Compare To Constant  Commented=on  relop=<=  const=sourceAccuracy  OutDataTypeStr=boolean
  Gain : Gain  Gain=1/distError
  Stop Simulation : Stop  Commented=on
  Subtract : Sum  Inputs=+-
  To Workspace1 : ToWorkspace  VariableName=ScoreL  SampleTime=-1
      settings: Save2DSignal=2-D array (concatenate along first dimension)
  wires:
  Data Store Read/1 -> Subtract/2
  Subtract/1 -> Distance/1
  Data Store Read2/1 -> Subtract/1
  Distance Threshold/1 -> Stop Simulation/1
  Distance/1 -> Gain/1, Distance Threshold/1
  Gain/1 -> To Workspace1/1

== system GradientAscent/Skill Scores/Source Estimate (SQ) ==
  Abs : Abs
  Constant1 : Constant  Value=MaxC
  Data Store Read : DataStoreRead  DataStoreName=Qest
  Divide : Product  Inputs=*/
  Q estimate : Subsystem
  Subtract1 : Sum  Inputs=-+
  To Workspace : ToWorkspace  VariableName=ScoreQ  SampleTime=-1
  wires:
  Divide/1 -> Abs/1
  Subtract1/1 -> Divide/1
  Abs/1 -> To Workspace/1
  Data Store Read/1 -> Subtract1/1
  Constant1/1 -> Divide/2, Subtract1/2

== system GradientAscent/Gradient Ascent/Goal Update/Goal Update ==
  In2 : Inport
  In3 : Inport  Port=2
  Enable : EnablePort
  Constant : Constant  Value=mag
  goalUpdate : MATLAB Function  TreatAsAtomicUnit=on
  Out2 : Outport  VectorParamsAs1DForOutWhenUnconnected=off
  wires:
  In3/1 -> goalUpdate/2(ang)
  goalUpdate/1(goal) -> Out2/1
  In2/1 -> goalUpdate/1(pose)
  Constant/1 -> goalUpdate/3(mag)

== system GradientAscent/Gradient Ascent/Goal Update/Goal Update Conditions ==
  In1 : Inport
  Data Store Read : DataStoreRead  DataStoreName=Peak
  Data Store Read1 : DataStoreRead  DataStoreName=angUpdate
  Data Store Read2 : DataStoreRead  DataStoreName=next
  Distance : Fcn  Expr=sqrt(u(1)^2+u(2)^2)
  Distance Threshold : simulink/Logic and Bit Operations/Compare To Constant  relop=<=  const=1.5  OutDataTypeStr=boolean
  Logical Operator : Logic  Operator=OR  AllPortsSameDT=off  OutDataTypeStr=boolean
  Logical Operator1 : Logic  Operator=OR  AllPortsSameDT=off  OutDataTypeStr=boolean
  Subtract : Sum  Inputs=+-
  Out1 : Outport  VectorParamsAs1DForOutWhenUnconnected=off
  wires:
  In1/1 -> Subtract/1
  Subtract/1 -> Distance/1
  Distance/1 -> Distance Threshold/1
  Distance Threshold/1 -> Logical Operator/2
  Data Store Read2/1 -> Logical Operator/1
  Logical Operator/1 -> Logical Operator1/1
  Data Store Read/1 -> Subtract/2
  Data Store Read1/1 -> Logical Operator1/2
  Logical Operator1/1 -> Out1/1

== system GradientAscent/Gradient Ascent/Goal Update/Initialize Goal ==
  In1 : Inport
  Constant : Constant  Value=init
  Data Store Read : DataStoreRead  DataStoreName=skip
  Data Store Read1 : DataStoreRead  DataStoreName=finalPoint
  Data Store Read2 : DataStoreRead  DataStoreName=PeakEst
  Switch : Switch  Criteria=u2 > Threshold
  Switch1 : Switch  Criteria=u2 > Threshold
  goal : Outport  VectorParamsAs1DForOutWhenUnconnected=off
  wires:
  Data Store Read/1 -> Switch/2
  In1/1 -> Switch/1
  Constant/1 -> Switch/3
  Switch/1 -> Switch1/3
  Data Store Read1/1 -> Switch1/2
  Data Store Read2/1 -> Switch1/1
  Switch1/1 -> goal/1

== system GradientAscent/Gradient Ascent/Goal Update/Skip Conditions ==
  In1 : Inport
  Constant1 : Constant
  Counter : dspswit3/Counter  Direction=Up  CountEvent=Rising edge  CounterSize=User defined  MaxCount=255  InitialCount=0  Output=Count  HitValue=32  ResetInput=off  SamplesPerFrame=1  Ts=1  CntDtype=double  HitDtype=Logical
  Data Store Write4 : DataStoreWrite  DataStoreName=skip
  Ground1 : Ground
  Switch1 : Switch  Criteria=u2 > Threshold
  wires:
  Constant1/1 -> Switch1/1
  Counter/1 -> Switch1/2
  Switch1/1 -> Data Store Write4/1
  Ground1/1 -> Switch1/3
  In1/1 -> Counter/1

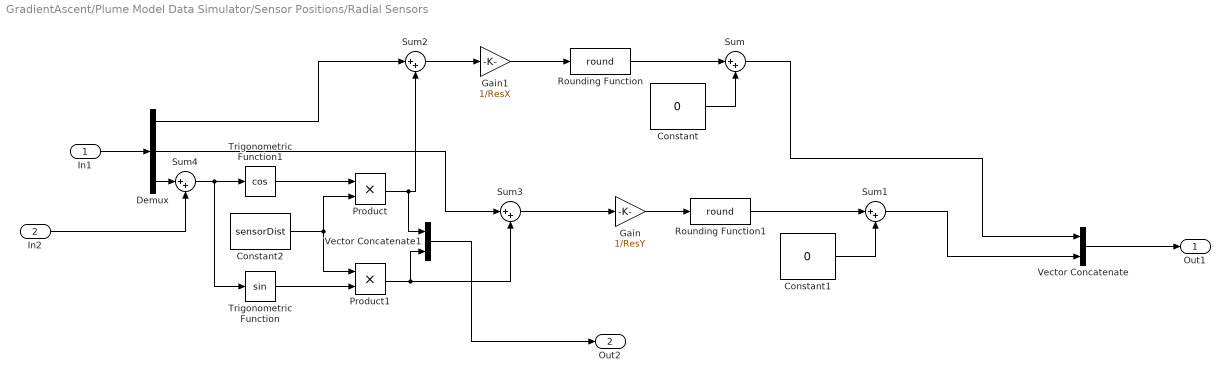
== system GradientAscent/Plume Model Data Simulator/Sensor Positions/Radial Sensors ==
  In1 : Inport
  In2 : Inport  Port=2
  Constant : Constant  Value=0
  Constant1 : Constant  Value=0
  Constant2 : Constant  Value=sensorDist
  Demux : Demux  Outputs=3
  Gain : Gain  Gain=1/ResY
  Gain1 : Gain  Gain=1/ResX
  Product : Product
  Product1 : Product
  Rounding Function : Rounding  Operator=round
  Rounding Function1 : Rounding  Operator=round
  Sum{,1..4} (5 alike) : Sum  Inputs=|++
  Trigonometric Function : Trigonometry
  Trigonometric Function1 : Trigonometry  Operator=cos
  Vector Concatenate : Concatenate
  Vector Concatenate1 : Concatenate
  Out1 : Outport  VectorParamsAs1DForOutWhenUnconnected=off
  Out2 : Outport  Port=2  VectorParamsAs1DForOutWhenUnconnected=off
  wires:
  Product/1 -> Vector Concatenate1/1, Sum2/2
  Sum2/1 -> Gain1/1
  Vector Concatenate/1 -> Out1/1
  Sum4/1 -> Trigonometric Function/1, Trigonometric Function1/1
  Demux/1 -> Sum2/1
  Vector Concatenate1/1 -> Out2/1
  Trigonometric Function/1 -> Product1/2
  In1/1 -> Demux/1
  Product1/1 -> Vector Concatenate1/2, Sum3/2
  In2/1 -> Sum4/2
  Constant1/1 -> Sum1/2
  Rounding Function1/1 -> Sum1/1
  Sum3/1 -> Gain/1
  Gain1/1 -> Rounding Function/1
  Gain/1 -> Rounding Function1/1
  Rounding Function/1 -> Sum/1
  Constant/1 -> Sum/2
  Sum/1 -> Vector Concatenate/1
  Sum1/1 -> Vector Concatenate/2
  Trigonometric Function1/1 -> Product/1
  Demux/3 -> Sum4/1
  Demux/2 -> Sum3/1
  Constant2/1 -> Product1/1, Product/2

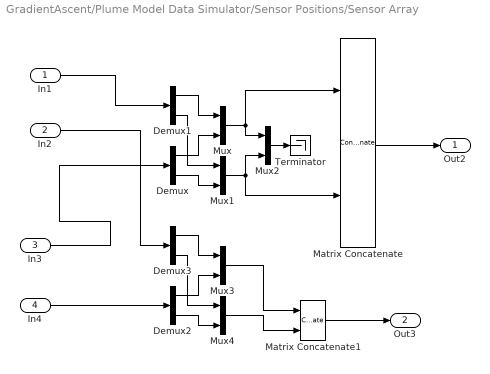
== system GradientAscent/Plume Model Data Simulator/Sensor Positions/Sensor Array ==
  In1 : Inport
  In2 : Inport  Port=2
  In3 : Inport  Port=3
  In4 : Inport  Port=4
  Demux{,1..3} (4 alike) : Demux  Outputs=2
  Matrix Concatenate : Concatenate  Mode=Multidimensional array  ConcatenateDimension=2
  Matrix Concatenate1 : Concatenate  Mode=Multidimensional array  ConcatenateDimension=2
  Mux{,1..4} (5 alike) : Mux  Inputs=2
  Terminator : Terminator
  Out2 : Outport  VectorParamsAs1DForOutWhenUnconnected=off
  Out3 : Outport  Port=2  VectorParamsAs1DForOutWhenUnconnected=off
  wires:
  Mux2/1 -> Terminator/1
  In1/1 -> Demux1/1
  Demux1/1 -> Mux/1
  Demux/1 -> Mux/2
  Demux1/2 -> Mux1/1
  Demux/2 -> Mux1/2
  Mux/1 -> Matrix Concatenate/1, Mux2/1
  Mux1/1 -> Mux2/2, Matrix Concatenate/2
  Matrix Concatenate/1 -> Out2/1
  Matrix Concatenate1/1 -> Out3/1
  In2/1 -> Demux3/1
  Demux3/1 -> Mux3/1
  Demux2/1 -> Mux3/2
  Demux3/2 -> Mux4/1
  Demux2/2 -> Mux4/2
  In4/1 -> Demux2/1
  Mux3/1 -> Matrix Concatenate1/1
  Mux4/1 -> Matrix Concatenate1/2
  In3/1 -> Demux/1

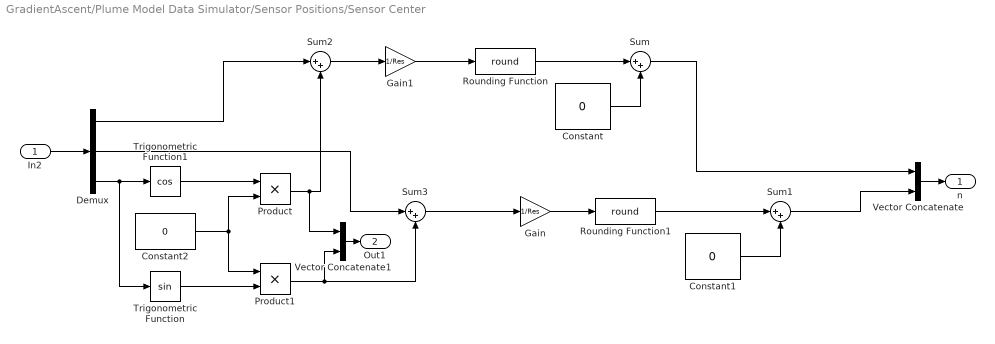
== system GradientAscent/Plume Model Data Simulator/Sensor Positions/Sensor Center ==
  In2 : Inport
  Constant : Constant  Value=0
  Constant1 : Constant  Value=0
  Constant2 : Constant  Value=0
  Demux : Demux  Outputs=3
  Gain : Gain  Gain=1/Res
  Gain1 : Gain  Gain=1/Res
  Product : Product
  Product1 : Product
  Rounding Function : Rounding  Operator=round
  Rounding Function1 : Rounding  Operator=round
  Sum{,1..3} (4 alike) : Sum  Inputs=|++
  Trigonometric Function : Trigonometry
  Trigonometric Function1 : Trigonometry  Operator=cos
  Vector Concatenate : Concatenate
  Vector Concatenate1 : Concatenate
  n : Outport  VectorParamsAs1DForOutWhenUnconnected=off
  Out1 : Outport  Port=2  VectorParamsAs1DForOutWhenUnconnected=off
  wires:
  Rounding Function/1 -> Sum/1
  Rounding Function1/1 -> Sum1/1
  Constant/1 -> Sum/2
  Constant1/1 -> Sum1/2
  Sum/1 -> Vector Concatenate/1
  Sum1/1 -> Vector Concatenate/2
  Gain1/1 -> Rounding Function/1
  Gain/1 -> Rounding Function1/1
  Sum2/1 -> Gain1/1
  Sum3/1 -> Gain/1
  In2/1 -> Demux/1
  Demux/1 -> Sum2/1
  Demux/2 -> Sum3/1
  Demux/3 -> Trigonometric Function/1, Trigonometric Function1/1
  Constant2/1 -> Product1/1, Product/2
  Product/1 -> Vector Concatenate1/1, Sum2/2
  Product1/1 -> Vector Concatenate1/2, Sum3/2
  Vector Concatenate/1 -> n/1
  Trigonometric Function1/1 -> Product/1
  Trigonometric Function/1 -> Product1/2
  Vector Concatenate1/1 -> Out1/1

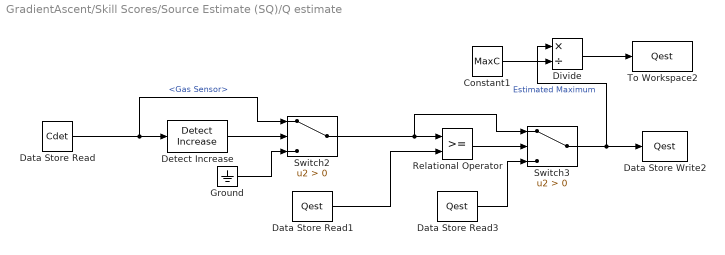
== system GradientAscent/Skill Scores/Source Estimate (SQ)/Q estimate ==
  Constant1 : Constant  Value=MaxC
  Data Store Read : DataStoreRead  DataStoreName=Cdet
  Data Store Read1 : DataStoreRead  DataStoreName=Qest
  Data Store Read3 : DataStoreRead  DataStoreName=Qest
  Data Store Write2 : DataStoreWrite  DataStoreName=Qest
  Detect Increase : simulink/Logic and Bit Operations/Detect Increase  vinit=0.0  OutDataTypeStr=boolean
  Divide : Product  Inputs=*/
  Ground : Ground
  Relational Operator : RelationalOperator  OutDataTypeStr=boolean  RndMeth=Simplest
  Switch2 : Switch  Criteria=u2 > Threshold
  Switch3 : Switch  Criteria=u2 > Threshold
  To Workspace2 : ToWorkspace  VariableName=Qest  SaveFormat=Timeseries  SampleTime=-1
  wires:
  Ground/1 -> Switch2/3
  Detect Increase/1 -> Switch2/2
  Relational Operator/1 -> Switch3/2
  Switch2/1 -> Switch3/1, Relational Operator/1
  Data Store Read3/1 -> Switch3/3
  Switch3/1 -> Divide/1, Data Store Write2/1  "Estimated Maximum"
  Data Store Read1/1 -> Relational Operator/2
  Data Store Read/1 -> Switch2/1, Detect Increase/1  "<Gas Sensor>"
  Constant1/1 -> Divide/2
  Divide/1 -> To Workspace2/1

== matlab function GradientAscent/Odometry Subscriber/Odom Conversion/Conversion ==
  data: yaw output; x input; y input; z input; w input
function yaw  = quat2eul(x,y,z,w)
%#codegen

% Convert the quaternion to a yaw angle (zyx euler angle)
eul = quat2eul([w,x,y,z]);
yaw = eul(1);

end

== matlab function GradientAscent/Plume Model Data Simulator/Static Plume Concentrations/MATLAB Function ==
  data: PlumeD input; Plume output; Peak output; OffsetY input
function [Plume, Peak] = fcn(PlumeD,OffsetY)

%Plume = squeeze(PlumeD(:,:,u));

%Plume = PlumeD(:,:,u);
Plume = PlumeD(:,:);

Cmax = max(max(Plume(:)));

Peak = [1 OffsetY+1];

end

function coord = maxmat( c )
as=size(c);
total_ele=numel(c);
[~,I]=max(c(:));
r=rem(I,as(1));
a=r;
b=((I-a)/as(1))+1;
if a==0
    a=as(1);
    b=b-1;
else
    a=r;
    b=b;
end

coord = [b,a]

end

== matlab function GradientAscent/Gradient Ascent/Goal Update/Goal Update/goalUpdate ==
  data: pose input; goal output; ang input; mag input
function goal  = fcn(pose, ang, mag)

xgoal = pose(1) + mag*cos(ang);
ygoal = pose(2) + mag*sin(ang);

xgoal = round(xgoal);
ygoal = round(ygoal);

goal = [xgoal,ygoal];

== matlab function GradientAscent/Gradient Ascent/GradAscent ==
  data: C input size=N+1; n input; ang output; N input; r input
function ang   = fcn(C,n,N,r)

fx = 0;
fy = 0;
Df = [];
n = n';

% calculate the gradient at vehicle center:
for i = 2:(N+1)
    fx = fx + (C(i)-C(1))*(n(1,i))/r;
    fy = fy + (C(i)-C(1))*(n(2,i))/r;
end

fx = fx/N;
fy = fy/N;
gradf = [fx,fy];
normf = norm(gradf);

% calculate directional derivative in each search direction:
for theta = 0:(2*pi/N):2*pi
    u = [cos(theta),sin(theta)];
    Du = gradf(1)*u(1) + gradf(2)*u(2);
    Df = [Df;Du];
end

% Select the largest directional derivative and compute the heading angle
% adjustment:
Df = Df/normf;
D = find(Df == max(Df(:)));
%d = max(setdiff(Df(:),max(Df(:))));

%ang = ((pi/4)*(D(1)-1));


if isempty(D)
    ang = pi;
else
    ang = ((pi/4)*(D(1)-1));
end
%}

== matlab function GradientAscent/Plume Model Data Simulator/Sensor Data Matrix/MATLAB Function ==
  data: plume input; cMap input; poses input; N input; Cdata data_store_memory size=[(N+1) 1]; Cdata1 output size=N+1; offY input; cMap1 output; maxPose data_store_memory size=2; MaxPose output size=2
function [Cdata1,cMap1,MaxPose]= fcn(plume,cMap,poses,N,offY)

Cdata = zeros(N,1);
Cdata1 = zeros(N,1);
cMap1 = zeros(size(plume,1),size(plume,2));

%coder.varsize('maxPose');
%Phi = PhiInput;
MaxPose = zeros(2,1);
maxPose = zeros(2,1);

for i = 1:N
    if poses(i,1) < 1
    poses(i,1) = 1;
    elseif poses(i,2) == 0
    poses(i,2) = 1;
    end

    cols = plume(:,poses(i,1));
    rows = cols(poses(i,2)+offY,1);
    
    Cdata(i) = rows(1);
    cMap(poses(i,2)+offY,poses(i,1)) = rows(1);
    
end

    cMap1 = cMap(:,:);
    Cdata1 = Cdata;
    
    p = find(Cdata1 == max(Cdata1));
    
    if size(p,1) == 1 
        %if size(poses,1) > 1
            maxPose(:,:) = [poses(p,1); poses(p,2)];
            %maxPose(1) = poses(p,1);
            %maxPose(2) = poses(p,2);
        %end
    else
        maxPose = [poses(1,1); poses(1,2)];
        %maxPose = [1; 1];
    end
    
    MaxPose = maxPose;

end
